simulink model "crusie_control"  (R2020a)
settings: Solver=ode45  StartTime=0.0  StopTime=120  RelTol=1e-3
undefined symbols (not defined in the file): b, m
settings Model: DataDictionary=varables.sldd  Creator=Jake  LastModifiedBy=Jake
settings DataIOCC: SaveOutput=off  SaveTime=off

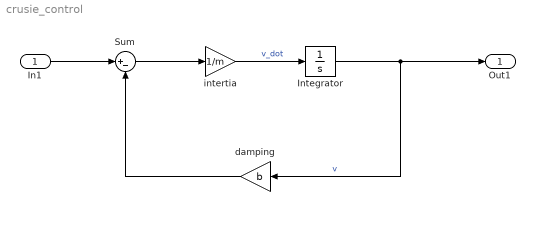
== system crusie_control ==
  In1 : Inport  OutDataTypeStr=double  PortDimensions=1  SampleTime=0
  Integrator : Integrator
  Sum : Sum  Inputs=|+-
  damping : Gain  Gain=b
  intertia : Gain  Gain=1/m
  Out1 : Outport  OutDataTypeStr=double  PortDimensions=1  SampleTime=0
  wires:
  damping/1 -> Sum/2
  intertia/1 -> Integrator/1  "v_dot"
  Integrator/1 -> damping/1, Out1/1  "v"
  In1/1 -> Sum/1
  Sum/1 -> intertia/1
